simulink model "unt53"  (R2017b)
settings: Solver=VariableStepAuto  StartTime=0.0  StopTime=1000  RelTol=1e-3
values from neighbouring files (symbols this model uses):
  kd = 1    [project_2023_12_25_P121_1.m]
  ki = 0.5    [project_2023_12_25_P121_1.m]
undefined symbols (not defined in the file or in its folder): kp
libraries: simulink x1
settings Model: Creator=Administrator  LastModifiedBy=Administrator

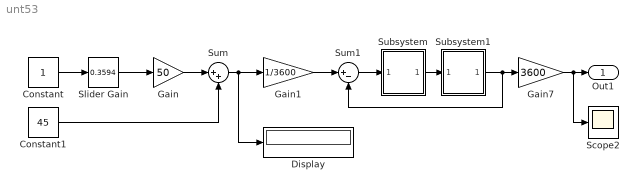
== system unt53 ==
  Constant : Constant
  Constant1 : Constant  Value=45
  Display : Display
  Gain : Gain  Gain=50
  Gain1 : Gain  Gain=1/3600
  Gain7 : Gain  Gain=3600
  Scope2 : Scope
  Slider Gain : simulink/Math Operations/Slider Gain  gain=0.3594  low=0  high=2
  Subsystem : Subsystem
  Subsystem1 : Subsystem
  Sum : Sum  Inputs=|++
  Sum1 : Sum  Inputs=|+-
  Out1 : Outport  SignalName=y
  wires:
  Constant1/1 -> Sum/2
  Sum/1 -> Display/1, Gain1/1
  Slider Gain/1 -> Gain/1
  Gain/1 -> Sum/1
  Constant/1 -> Slider Gain/1
  Gain1/1 -> Sum1/1
  Sum1/1 -> Subsystem/1(In1)
  Subsystem/1(Out1) -> Subsystem1/1(In1)
  Subsystem1/1(Out1) -> Sum1/2, Gain7/1
  Gain7/1 -> Scope2/1, Out1/1

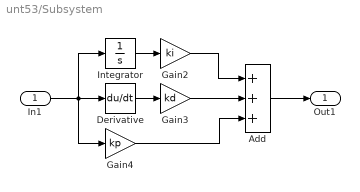
== system unt53/Subsystem ==
  In1 : Inport
  Add : Sum  Inputs=+++
  Derivative : Derivative
  Gain2 : Gain  Gain=ki
  Gain3 : Gain  Gain=kd
  Gain4 : Gain  Gain=kp
  Integrator : Integrator
  Out1 : Outport
  wires:
  Derivative/1 -> Gain3/1
  In1/1 -> Gain4/1, Derivative/1, Integrator/1
  Gain3/1 -> Add/2
  Integrator/1 -> Gain2/1
  Gain2/1 -> Add/1
  Gain4/1 -> Add/3
  Add/1 -> Out1/1

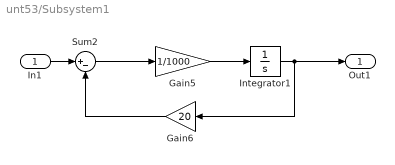
== system unt53/Subsystem1 ==
  In1 : Inport
  Gain5 : Gain  Gain=1/1000
  Gain6 : Gain  Gain=20
  Integrator1 : Integrator
  Sum2 : Sum  Inputs=|+-
  Out1 : Outport
  wires:
  Sum2/1 -> Gain5/1
  In1/1 -> Sum2/1
  Integrator1/1 -> Out1/1, Gain6/1
  Gain6/1 -> Sum2/2
  Gain5/1 -> Integrator1/1
